simulink model "motion_planning"  (R2019b)
settings: Solver=ode1  StartTime=0.0  StopTime=10  FixedStep=0.001  RelTol=1e-3
undefined symbols (not defined in the file): __PRM__SERIALIZED__DATA__, SubsystemReferenceBlock, wayPoints_trajectory
libraries: robotcorelib x3, robotmaniplib x2, simulink x1, sm_lib x1
settings Model: Creator=Robot  LastModifiedBy=Robot
settings ExplorerConfigSet: InternalSimMechanicsExplorerSettings="<ExplorerConfiguration><canonicalview>default</canonicalview><AnimationSetting><BasePlaybackSpeed>1.0</BasePlaybackSpeed><PlaybackSpeedFactor>0.5</PlaybackSpeedFactor></AnimationSetting><TilePanel><TileInfo><Tiles Columns=\"2\" Count=\"4\" Rows=\"2\"><Column Weight=\"0.5\"/><Column Weight=\"0.5\"/><Row Weight=\"0.4994\"/><Row Weight=\"0.5006\"/><Tile Height=\"1\" Width=\"1\" X=\"0\" Y=\"0\"/><Tile Height=\"1\" Width=\"1\" X=\"0\" Y=\"1\"/><Tile Height=\"1\" Width=\"1\" X=\"1\" Y=\"0\"/><Tile Height=\"1\" Width=\"1\" X=\"1\" Y=\"1\"/></Tiles></TileInfo><SceneInfo><SceneViewer><BGColor><R>0.60000002384185791</R><G>0.60000002384185791</G><B>0.60000002384185791</B></BGColor><Camera><DoPerspective>off</DoPerspective><Position><X>0.5939565506279334</X><Y>-0.593956547369122512</Y><Z>0.623546953554225181</Z></Position><Center><X>0.0166062814383075297</X><Y>-0.0166062781794966419</Y><Z>0.0461966843645992969</Z></Center><Up><X>-0.408248290463863073</X><Y>0.408248290463863073</Y><Z>0.816496580927726145</Z></Up><ViewLimDist>1</ViewLimDist><YLim>0.29553410034955091</YLim><XLim>0.436991995573043857</XLim></Camera></SceneViewer><SceneViewer><BGColor><R>0.60000002384185791</R><G>0.60000002384185791</G><B>0.60000002384185791</B></BGColor><Camera><DoPerspective>off</DoPerspective><Position><X>9.57470331838794486e-09</X><Y>-6.31589205934979248e-09</Y><Z>1.13676420859947735</Z></Position><Center><X>9.57470331838794486e-09</X><Y>-6.31589205934979248e-09</Y><Z>0.136764208599477355</Z></Center><Up><X>0</X><Y>1</Y><Z>-0</Z></Up><ViewLimDist>1</ViewLimDist><YLim>0.309000012278556835</YLim><XLim>0.455878941881817046</XLim></Camera></SceneViewer><SceneViewer><BGColor><R>0.60000002384185791</R><G>0.60000002384185791</G><B>0.60000002384185791</B></BGColor><Camera><DoPerspective>off</DoPerspective><Position><X>1.00000000957470325</X><Y>-6.31589203159421686e-09</Y><Z>0.136764447018056456</Z></Position><Center><X>9.57470325246845277e-09</X><Y>-6.31589203159421686e-09</Y><Z>0.136764447018056456</Z></Center><Up><X>-0</X><Y>0</Y><Z>1</Z></Up><ViewLimDist>1</ViewLimDist><YLim>0.20897417243762581</YLim><XLim>0.309000012278556835</XLim></Camera></SceneViewer><SceneViewer><BGColor><R>0.60000002384185791</R><G>0.60000002384185791</G><B>0.60000002384185791</B></BGColor><Camera><DoPerspective>off</DoPerspective><Position><X>0.593956539594466926</X><Y>-0.593956536335656149</Y><Z>0.623546933057384845</Z></Position><Center><X>0.0166062704048410871</X><Y>-0.0166062671460303485</Y><Z>0.046196663867759058</Z></Center><Up><X>-0.408248290463863073</X><Y>0.408248290463863073</Y><Z>0.816496580927726145</Z></Up><ViewLimDist>1</ViewLimDist><YLim>0.296198221923370142</YLim><XLim>0.436991995573043857</XLim></Camera></SceneViewer></SceneInfo></TilePanel><MechEditorPanel><Cameras/><GfxPanelCameraMap/><VideoCreator><PlaybackSpeedRatio>1.0</PlaybackSpeedRatio><FrameRate>30</FrameRate><VideoFormat>Motion JPEG AVI</VideoFormat><FrameSize>auto</FrameSize></VideoCreator></MechEditorPanel></ExplorerConfiguration>"

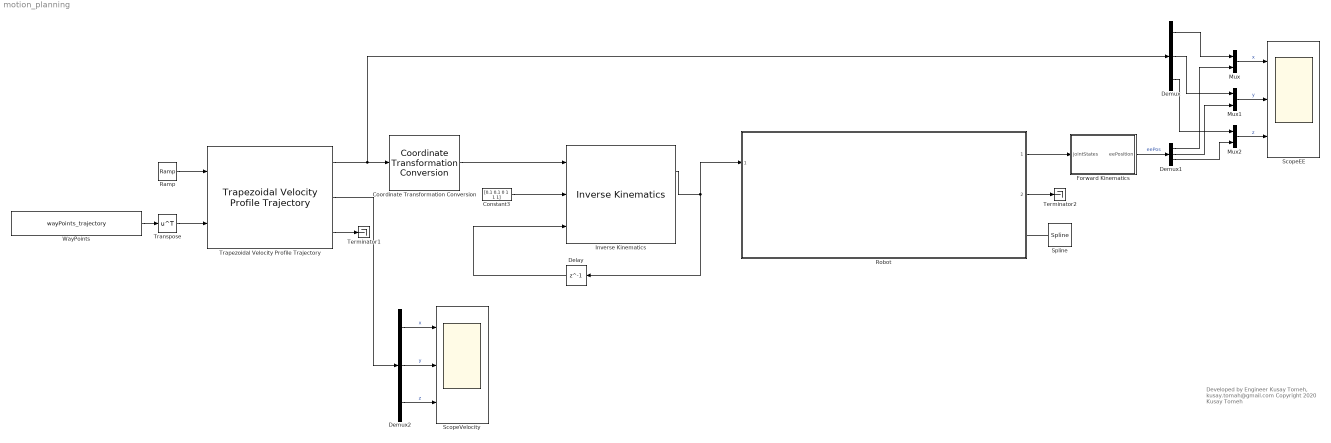
== system motion_planning ==
  note: Developed by Engineer Kusay Tomeh,
      | kusay.tomah@gmail.com
      | Copyright 2020 Kusay Tomeh
  Constant3 : Constant  Value=[0.1 0.1 0 1 1 1]  VectorParams1D=off
  Coordinate Transformation Conversion : robotcorelib/Coordinate Transformation Conversion  InputRepresentation=Translation Vector  InputEulerSequence=ZYX  ShowTrVecInputPort=on  OutputRepresentation=Homogeneous Transformation  OutputEulerSequence=ZYX  ShowTrVecOutputPort=on  SimulateUsing=Interpreted execution
      settings: SourceProductBaseCode=RO
  Delay : Delay  DelayLength=1
  Demux : Demux  Outputs=3
  Demux1 : Demux  Outputs=3
  Demux2 : Demux  Outputs=3
  Forward Kinematics : Subsystem
  Inverse Kinematics : robotmaniplib/Inverse Kinematics  RigidBodyTree=robot  EndEffector=end_effector  ShowInfo=off  SolverName=BFGS Gradient Projection  EnforceJointLimits=on  MaxIterations=1500  MaxTime=10  GradientTolerance=1e-7  SolutionTolerance=1e-6  StepTolerance=1e-14  ErrorChangeTolerance=1e-12  UseErrorDamping=on  DampingBias=0.0025  SimulateUsing=Interpreted execution
      settings: SourceProductName=Robotics System Toolbox
  Mux : Mux  Inputs=2
  Mux1 : Mux  Inputs=2
  Mux2 : Mux  Inputs=2
  Ramp : simulink/Sources/Ramp  slope=1  start=1  InitialOutput=0
  Robot : Subsystem  BlockKeywords=__PRM__SERIALIZED__DATA__:SubsystemReferenceBlock  ReferencedSubsystem=RobotModelWithFloor
  ScopeEE : Scope  NumInputPorts=3
  ScopeVelocity : Scope  NumInputPorts=3
  Spline : sm_lib/Curves and Surfaces/Spline  GraphicAmbientColor=[0.15 0.15 0.15 1.0]  GraphicDiffuseColor=[1.0 0.0 0.0]  DataPoints=wayPoints_trajectory  DataPointsUnits=m  GraphicEmissiveColor=[0.0 0.0 0.0 1.0]  EndConditionType=Closed  MarkerShape=Sphere  MarkerSize=10  GraphicType=FromGeometry  GraphicOpacity=1  GraphicShininess=100  GraphicSpecularColor=[0.5 0.5 0.5 1.0]  GraphicVisPropType=SimpleVisualProperties
      settings: SourceProductName=Simscape Multibody
  Terminator1 : Terminator
  Terminator2 : Terminator
  Transpose : Math  Operator=transpose  SignedPower=off  SaturateOnIntegerOverflow=on
  Trapezoidal Velocity Profile Trajectory : robotcorelib/Trapezoidal Velocity Profile Trajectory  WaypointSource=External  Waypoints=[ 0, -0.5, -1; 0, 0.5, 1 ]  NumParams=0  Parameter1=End Time  Parameter2=End Time  ParameterSource=External  PeakVelocity=[ 1; 1; 1 ]  Acceleration=[ 1; 2 ]  EndTime=[ 1; 1; 1 ]  AccelTime=[ 1; 2 ]  SimulateUsing=Interpreted execution
      settings: SourceProductName=Robotics System Toolbox  SourceProductBaseCode=RO
  WayPoints : Constant  Value=wayPoints_trajectory  SampleTime=-1
  wires:
  Inverse Kinematics/1 -> Robot/1, Delay/1
  Robot/1 -> Forward Kinematics/1(jointStates)
  Coordinate Transformation Conversion/1 -> Inverse Kinematics/1
  Trapezoidal Velocity Profile Trajectory/1 -> Demux/1, Coordinate Transformation Conversion/1
  Constant3/1 -> Inverse Kinematics/2
  Forward Kinematics/1(eePosition) -> Demux1/1  "eePos"
  Mux/1 -> ScopeEE/1  "x"
  Mux1/1 -> ScopeEE/2  "y"
  Mux2/1 -> ScopeEE/3  "z"
  Demux/1 -> Mux/1
  Demux/2 -> Mux1/1
  Demux/3 -> Mux2/1
  Demux1/1 -> Mux/2
  Demux1/2 -> Mux1/2
  Demux1/3 -> Mux2/2
  Ramp/1 -> Trapezoidal Velocity Profile Trajectory/1
  Delay/1 -> Inverse Kinematics/3
  Transpose/1 -> Trapezoidal Velocity Profile Trajectory/2
  WayPoints/1 -> Transpose/1
  Trapezoidal Velocity Profile Trajectory/2 -> Demux2/1
  Trapezoidal Velocity Profile Trajectory/3 -> Terminator1/1
  Robot/2 -> Terminator2/1
  Demux2/2 -> ScopeVelocity/2  "y"
  Demux2/1 -> ScopeVelocity/1  "x"
  Demux2/3 -> ScopeVelocity/3  "z"
  connections:
  Spline/LConn1 -- Robot/RConn1

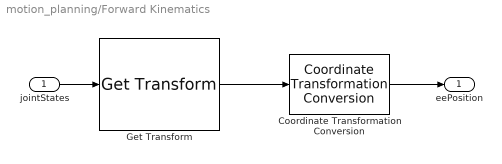
== system motion_planning/Forward Kinematics ==
  jointStates : Inport
  Coordinate Transformation Conversion : robotcorelib/Coordinate Transformation Conversion  InputRepresentation=Homogeneous Transformation  InputEulerSequence=ZYX  ShowTrVecInputPort=on  OutputRepresentation=Translation Vector  OutputEulerSequence=ZYX  ShowTrVecOutputPort=on  SimulateUsing=Code generation
      settings: SourceProductBaseCode=RO
      settings: AttributesFormatString=|
      | %<InputRepresentation>
      | to %<OutputRepresentation>
  Get Transform : robotmaniplib/Get Transform  RigidBodyTree=robot  SourceBody=end_effector  TargetBody=world  SimulateUsing=Interpreted execution
      settings: SourceProductName=Robotics System Toolbox
  eePosition : Outport  VectorParamsAs1DForOutWhenUnconnected=off
  wires:
  jointStates/1 -> Get Transform/1
  Coordinate Transformation Conversion/1 -> eePosition/1
  Get Transform/1 -> Coordinate Transformation Conversion/1
